simulink model "sampleModel1490"  (R2023a)
settings: Solver=VariableStepAuto  StartTime=0.0  StopTime=10.0  RelTol=1e-3
libraries: hdlsllib x5
settings Model: Creator=user1  LastModifiedBy=user1

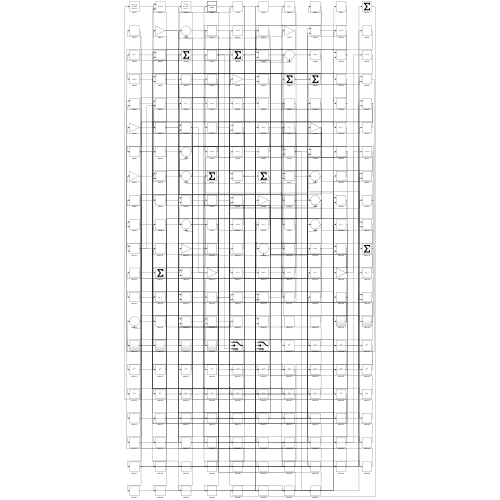
[thumbnail: Simulink's stored preview of the top-level diagram]
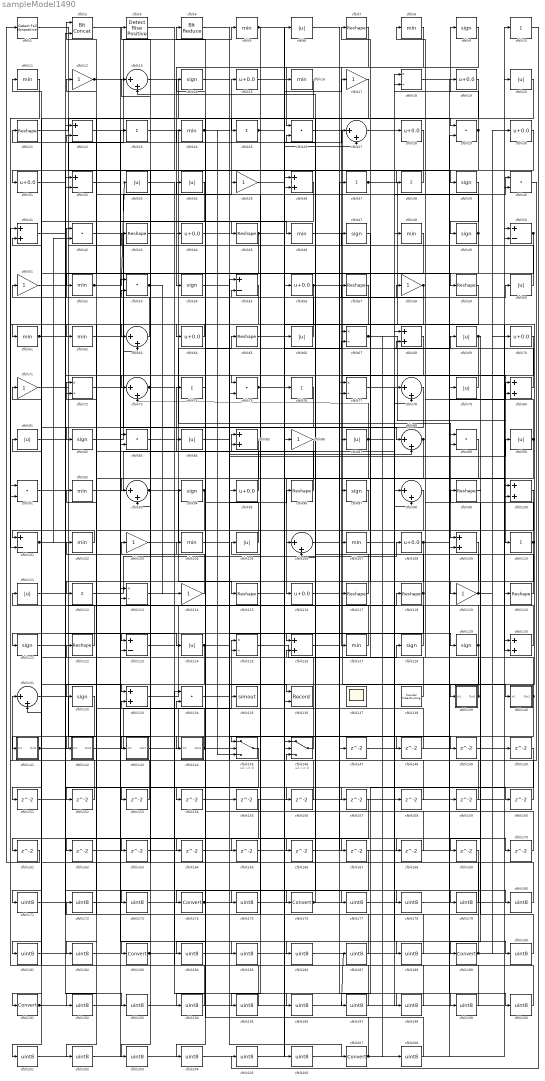
== system sampleModel1490 ==
  cfblk1 : hdlsllib/Logic and Bit Operations/Detect Fall Nonpositive  vinit=0  OutDataTypeStr=boolean
  cfblk{10,23,25,37..38,74,76,110,112} (9 alike) : Sum  Inputs=+
  cfblk{36,41,68,80,85,100,109,126,130,133} (10 alike) : Sum
  cfblk{22,32,50,55,101,123} (6 alike) : Sum  Inputs=+-
  cfblk{5,8,11,16,24,46,48,52,61..62,92,102,104,107,127} (15 alike) : MinMax
  cfblk{12,17,35,51,58,71,86,103,114,119} (10 alike) : Gain
  cfblk{6,20,33..34,60,66,69,79,81,84,87,90,105,111,124} (15 alike) : Abs  SaturateOnIntegerOverflow=off
  cfblk{13,27,63,73,78,88,93,98,106,131} (10 alike) : Sum  Inputs=|++
  cfblk{15,19,28,30..31,44,56,64,70,95,108,116} (12 alike) : Bias  Bias=0.0  SaturateOnIntegerOverflow=off
  cfblk{18,67,72,77,113,125} (6 alike) : Product  Inputs=*/  RndMeth=Zero  SaturateOnIntegerOverflow=on
  cfblk{7,21,43,45,57,59,65,96,99,115,117..118,120,122} (14 alike) : Reshape
  cfblk{9,14,39,47,49,54,82,94,97,121,128..129,132} (13 alike) : Signum
  cfblk{26,29,40,42,53,75,83,89,91,134} (10 alike) : DotProduct  OutDataTypeStr=Inherit: Inherit via internal rule
  cfblk135 : ToWorkspace  VariableName=simout  SaveFormat=Timeseries  SampleTime=-1
  cfblk136 : Record  FileSettingsInternal="{\"entries\":[{\"content\":{\"excelSettings\":{\"content\":{},\"type\":\"Streamout.ExcelSettings\"}},\"type\":\"Streamout.FileSettingStorage\",\"uuid\":\"\"}],\"packageUris\":[\"http:\\/\\/schema.mathworks.com\\/mf0\\/streamout_blocks\\/R2020a\"],\"version\":\"1.0\"}"  Layout=[1 1]  SignalsInternal="{\"entries\":[{\"content\":{\"signals\":[{\"content\":{\"blockPath\":[],\"dimensions\":[1],\"domain\":\"\",\"lineColor\":\"#a2142f\",\"plots\":[1],\"port\":1,\"signalID\":1211,\"signalName\":\"XY Graph:1\"},\"type\":\"RecordBlkView.Signal\",\"uuid\":\"\"},{\"content\":{\"blockPath\":[],\"dimensions\":[1],\"domain\":\"\",\"lineColor\":\"#139fff\",\"plots\":[1],\"port\":2,\"signalID\":1214,\"signalName\":\"XY Graph:2\"},\"type\":\"RecordBlkView.Signal\",\"uuid\":\"\"}]},\"type\":\"RecordBlkView.InputSignals\",\"uuid\":\"\"}],\"packageUris\":[\"http:\\/\\/schema.mathworks.com\\/mf0\\/streamout_blocks\\/R2020a\"],\"version\":\"1.0\"}"  VisualizationBindings="{\"xyplotplugin\":{\"info\":[{\"series\":[{\"bindingParametersList\":[{\"parameter\":\"X-Axis\",\"signalID\":1211,\"signalName\":\"XY Graph:1\"},{\"parameter\":\"Y-Axis\",\"signalID\":1214,\"signalName\":\"XY Graph:2\"}],\"seriesID\":2209}],\"subplotID\":1}]}}"  CompatibilityTag=XY  st=-1
  cfblk137 : Scope
      settings: Floating=on
  cfblk138 : hdlsllib/Sources/Counter Free-Running  NumBits=16  tsamp=-1
  cfblk139 : Subsystem
      settings: LibrarySourceBlock=|
      | hdlsllib/Ports &
      | Subsystems/Subsystem
  cfblk140 : Subsystem
      settings: LibrarySourceBlock=|
      | hdlsllib/Ports &
      | Subsystems/Subsystem
  cfblk141 : Subsystem
      settings: LibrarySourceBlock=|
      | hdlsllib/Ports &
      | Subsystems/Subsystem
  cfblk142 : Subsystem
      settings: LibrarySourceBlock=|
      | hdlsllib/Ports &
      | Subsystems/Subsystem
  cfblk143 : Subsystem
      settings: LibrarySourceBlock=|
      | hdlsllib/Ports &
      | Subsystems/Subsystem
  cfblk144 : Subsystem
      settings: LibrarySourceBlock=|
      | hdlsllib/Ports &
      | Subsystems/Subsystem
  cfblk145 : Switch  SaturateOnIntegerOverflow=off  InputSameDT=off
  cfblk146 : Switch  SaturateOnIntegerOverflow=off  InputSameDT=off
  cfblk{147..170} (24 alike) : Delay  SampleTime=1
  cfblk{171..173,175,177..182,184..188,190,192..206,208} (32 alike) : DataTypeConversion  OutDataTypeStr=uint8  SaturateOnIntegerOverflow=off  RndMeth=Floor
  cfblk{174,176,183,189,191,207} (6 alike) : DataTypeConversion  SaturateOnIntegerOverflow=off  RndMeth=Floor
  cfblk2 : hdlsllib/Logic and Bit Operations/Bit Concat  numInputs=2
  cfblk3 : hdlsllib/Logic and Bit Operations/Detect Rise Positive  vinit=0  OutDataTypeStr=boolean
  cfblk4 : hdlsllib/Logic and Bit Operations/Bit Reduce  mode=AND
  wires:
  cfblk42/1 -> cfblk88/1
  cfblk23/1 -> cfblk109/1
  cfblk12/1 -> cfblk44/1, cfblk179/1
  cfblk52/1 -> cfblk33/1, cfblk160/1
  cfblk121/1 -> cfblk5/1
  cfblk67/1 -> cfblk110/1, cfblk208/1
  cfblk117/1 -> cfblk85/1
  cfblk133/1 -> cfblk118/1
  cfblk86/1 -> cfblk116/1
  cfblk7/1 -> cfblk54/1
  cfblk26/1 -> cfblk139/1(In1)
  cfblk46/1 -> cfblk140/1(In1)
  cfblk88/1 -> cfblk126/1, cfblk143/1(In1)
  cfblk29/1 -> cfblk9/1, cfblk163/1
  cfblk112/1 -> cfblk108/1
  cfblk93/1 -> cfblk115/1, cfblk185/1
  cfblk125/1 -> cfblk128/1
  cfblk82/1 -> cfblk15/1
  cfblk63/1 -> cfblk42/1
  cfblk44/1 -> cfblk95/1
  cfblk109/1 -> cfblk112/1
  cfblk8/1 -> cfblk127/1
  cfblk90/1 -> cfblk43/1, cfblk195/1
  cfblk62/1 -> cfblk97/1
  cfblk75/1 -> cfblk76/1, cfblk67/2
  cfblk47/1 -> cfblk117/1
  cfblk115/1 -> cfblk6/1
  cfblk21/1 -> cfblk29/1
  cfblk71/1 -> cfblk23/1
  cfblk39/1 -> cfblk49/1
  cfblk49/1 -> cfblk64/1, cfblk12/1
  cfblk64/1 -> cfblk62/1
  cfblk143/1(Out1) -> cfblk125/1
  cfblk141/1(Out1) -> cfblk68/1, cfblk170/1
  cfblk130/1 -> cfblk11/1
  cfblk140/1(Out1) -> cfblk102/1, cfblk7/1, cfblk145/2
  cfblk142/1(Out1) -> cfblk135/1
  cfblk55/1 -> cfblk123/1
  cfblk56/1 -> cfblk100/1, cfblk73/1
  cfblk119/1 -> cfblk57/1, cfblk70/1, cfblk85/2
  cfblk114/1 -> cfblk92/1
  cfblk4/1 -> cfblk88/2
  cfblk58/1 -> cfblk107/1, cfblk101/2, cfblk142/1(In1)
  cfblk9/1 -> cfblk26/1
  cfblk127/1 -> cfblk72/1
  cfblk40/1 -> cfblk131/1
  cfblk38/1 -> cfblk31/1
  cfblk103/1 -> cfblk65/1
  cfblk32/1 -> cfblk46/1
  cfblk17/1 -> cfblk52/1
  cfblk69/1 -> cfblk68/2, cfblk169/1
  cfblk131/1 -> cfblk144/1(In1)
  cfblk33/1 -> cfblk94/1
  cfblk37/1 -> cfblk130/2, cfblk19/1
  cfblk106/1 -> cfblk37/1
  cfblk79/1 -> cfblk4/1
  cfblk13/1 -> cfblk25/1
  cfblk80/1 -> cfblk58/1
  cfblk24/1 -> cfblk129/1, cfblk145/3, cfblk188/1
  cfblk99/1 -> cfblk189/1
  cfblk138/1 -> cfblk125/2
  cfblk102/1 -> cfblk101/1
  cfblk73/1 -> cfblk3/1, cfblk168/1
  cfblk104/1 -> cfblk207/1
  cfblk66/1 -> cfblk53/2
  cfblk95/1 -> cfblk74/1
  cfblk126/1 -> cfblk60/1
  cfblk5/1 -> cfblk45/1, cfblk145/1, cfblk67/1
  cfblk139/1(Out1) -> cfblk126/2, cfblk8/1
  cfblk59/1 -> cfblk63/1
  cfblk144/1(Out1) -> cfblk122/1, cfblk177/1
  cfblk96/1 -> cfblk2/1
  cfblk101/1 -> cfblk124/1, cfblk42/2
  cfblk20/1 -> cfblk176/1
  cfblk107/1 -> cfblk28/1
  cfblk25/1 -> cfblk17/1, cfblk75/1, cfblk39/1
  cfblk2/1 -> cfblk87/1
  cfblk108/1 -> cfblk80/1, cfblk192/1
  cfblk122/1 -> cfblk81/1
  cfblk124/1 -> cfblk132/1, cfblk90/1, cfblk96/1
  cfblk65/1 -> cfblk100/2
  cfblk28/1 -> cfblk32/2
  cfblk51/1 -> cfblk59/1
  cfblk72/1 -> cfblk63/2
  cfblk60/1 -> cfblk47/1
  cfblk100/1 -> cfblk106/1
  cfblk94/1 -> cfblk123/2, cfblk194/1
  cfblk68/1 -> cfblk82/1
  cfblk36/1 -> cfblk183/1
  cfblk129/1 -> cfblk55/2, cfblk131/2
  cfblk1/1 -> cfblk77/2
  cfblk48/1 -> cfblk191/1
  cfblk34/1 -> cfblk141/1(In1)
  cfblk16/1 -> cfblk174/1
  cfblk146/1 -> cfblk71/1
  cfblk70/1 -> cfblk72/2
  cfblk50/1 -> cfblk75/2, cfblk175/1
  cfblk61/1 -> cfblk165/1, cfblk166/1
  cfblk118/1 -> cfblk121/1, cfblk13/2
  cfblk35/1 -> cfblk27/1
  cfblk128/1 -> cfblk105/1
  cfblk91/1 -> cfblk133/1
  cfblk54/1 -> cfblk136/1
  cfblk87/1 -> cfblk73/2, cfblk40/1, cfblk182/1
  cfblk92/1 -> cfblk69/1
  cfblk19/1 -> cfblk61/1
  cfblk98/1 -> cfblk146/2
  cfblk120/1 -> cfblk21/1
  cfblk110/1 -> cfblk119/1, cfblk51/1
  cfblk11/1 -> cfblk91/2
  cfblk105/1 -> cfblk84/1
  cfblk45/1 -> cfblk27/2, cfblk151/1
  cfblk27/1 -> cfblk18/1
  cfblk53/1 -> cfblk93/1, cfblk114/1
  cfblk3/1 -> cfblk38/1
  cfblk6/1 -> cfblk147/1
  cfblk147/1 -> cfblk50/1
  cfblk14/1 -> cfblk148/1
  cfblk148/1 -> cfblk53/1
  cfblk43/1 -> cfblk149/1
  cfblk149/1 -> cfblk80/2
  cfblk151/1 -> cfblk2/2
  cfblk145/1 -> cfblk152/1
  cfblk152/1 -> cfblk91/1
  cfblk57/1 -> cfblk153/1
  cfblk153/1 -> cfblk32/1
  cfblk85/1 -> cfblk154/1
  cfblk154/1 -> cfblk130/1
  cfblk84/1 -> cfblk155/1
  cfblk123/1 -> cfblk156/1
  cfblk156/1 -> cfblk55/1
  cfblk81/1 -> cfblk157/1
  cfblk158/1 -> cfblk146/1
  cfblk159/1 -> cfblk93/2
  cfblk160/1 -> cfblk133/2
  cfblk76/1 -> cfblk161/1
  cfblk161/1 -> cfblk1/1
  cfblk97/1 -> cfblk162/1
  cfblk162/1 -> cfblk109/2
  cfblk163/1 -> cfblk13/1
  cfblk74/1 -> cfblk164/1
  cfblk164/1 -> cfblk77/1
  cfblk165/1 -> cfblk98/2
  cfblk166/1 -> cfblk106/2
  cfblk31/1 -> cfblk167/1
  cfblk168/1 -> cfblk146/3
  cfblk170/1 -> cfblk34/1
  cfblk78/1 -> cfblk171/1
  cfblk171/1 -> cfblk86/1
  cfblk169/1 -> cfblk172/1
  cfblk172/1 -> cfblk78/1
  cfblk30/1 -> cfblk173/1
  cfblk173/1 -> cfblk78/2
  cfblk174/1 -> cfblk136/2, cfblk204/1
  cfblk175/1 -> cfblk16/1
  cfblk176/1 -> cfblk26/2, cfblk79/1
  cfblk177/1 -> cfblk20/1
  cfblk111/1 -> cfblk178/1
  cfblk178/1 -> cfblk29/2
  cfblk179/1 -> cfblk111/1
  cfblk113/1 -> cfblk180/1
  cfblk180/1 -> cfblk103/1
  cfblk157/1 -> cfblk181/1
  cfblk181/1 -> cfblk113/1
  cfblk182/1 -> cfblk113/2
  cfblk183/1 -> cfblk40/2, cfblk98/1
  cfblk167/1 -> cfblk184/1
  cfblk184/1 -> cfblk36/1
  cfblk185/1 -> cfblk36/2
  cfblk22/1 -> cfblk186/1
  cfblk186/1 -> cfblk158/1
  cfblk187/1 -> cfblk22/1
  cfblk188/1 -> cfblk22/2
  cfblk189/1 -> cfblk35/1, cfblk30/1
  cfblk77/1 -> cfblk190/1
  cfblk190/1 -> cfblk99/1
  cfblk191/1 -> cfblk187/1, cfblk18/2, cfblk120/1
  cfblk192/1 -> cfblk48/1
  cfblk41/1 -> cfblk193/1
  cfblk193/1 -> cfblk150/1
  cfblk194/1 -> cfblk41/1
  cfblk195/1 -> cfblk41/2
  cfblk134/1 -> cfblk196/1
  cfblk196/1 -> cfblk50/2
  cfblk150/1 -> cfblk197/1
  cfblk197/1 -> cfblk134/1
  cfblk116/1 -> cfblk198/1
  cfblk198/1 -> cfblk134/2
  cfblk83/1 -> cfblk199/1
  cfblk199/1 -> cfblk14/1
  cfblk18/1 -> cfblk200/1
  cfblk200/1 -> cfblk83/1
  cfblk132/1 -> cfblk201/1
  cfblk201/1 -> cfblk83/2
  cfblk89/1 -> cfblk202/1
  cfblk202/1 -> cfblk66/1
  cfblk155/1 -> cfblk203/1
  cfblk203/1 -> cfblk89/1
  cfblk204/1 -> cfblk89/2
  cfblk10/1 -> cfblk205/1
  cfblk205/1 -> cfblk56/1
  cfblk15/1 -> cfblk206/1
  cfblk206/1 -> cfblk10/1
  cfblk207/1 -> cfblk159/1, cfblk24/1
  cfblk208/1 -> cfblk104/1

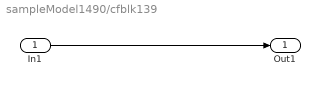
== system sampleModel1490/cfblk139 ==
  In1 : Inport
  Out1 : Outport
  wires:
  In1/1 -> Out1/1

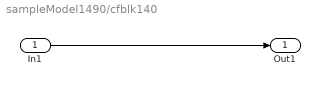
== system sampleModel1490/cfblk140 ==
  In1 : Inport
  Out1 : Outport
  wires:
  In1/1 -> Out1/1

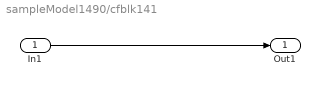
== system sampleModel1490/cfblk141 ==
  In1 : Inport
  Out1 : Outport
  wires:
  In1/1 -> Out1/1

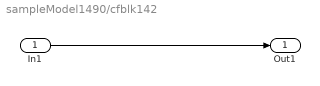
== system sampleModel1490/cfblk142 ==
  In1 : Inport
  Out1 : Outport
  wires:
  In1/1 -> Out1/1

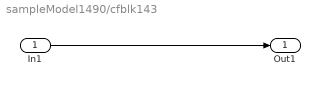
== system sampleModel1490/cfblk143 ==
  In1 : Inport
  Out1 : Outport
  wires:
  In1/1 -> Out1/1

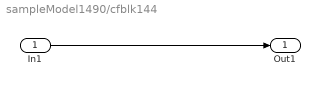
== system sampleModel1490/cfblk144 ==
  In1 : Inport
  Out1 : Outport
  wires:
  In1/1 -> Out1/1
